simulink library "SERGIOarm"  (Simulink 7.9)
settings: Solver=ode45  StartTime=0.0  StopTime=10.0  RelTol=1e-3
undefined symbols (not defined in the file or in its folder): DiscIntNeverNeededParam
settings Model: Creator=root  LastModifiedBy=root

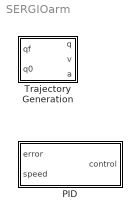
== system SERGIOarm ==
  PID : Subsystem  mask(PID Controller with anti wind-up){Kc=0, Ki=0, Kd=0, uplim=0, lowlim=0, Ts=0}
      mask prompts: Kc "P gain"; Ki "I gain"; Kd "D gain"; uplim "Integrator Upper Limit"; lowlim "Integrator Low Limit"; Ts "Sampling time (for integrator)"
      mask help: Outputs a control effort based on position error (error) and speed error (speed).
  Trajectory Generation : Subsystem  mask(Trajectory Generation){Vmax=0, Amax=0, dif_in=0}
      mask prompts: Vmax "Maximum Velocity"; Amax "Maximum Acceleration"; dif_in "Minimum Setpoint Change"
      mask help: Outputs setpoints (q) based on the starting point (q0) and end point (qf). The setpoints follow a fastest trajectory under the constraints of maximum velocity and maximum acceleration. Only outputs a trajectory if the setpoint change is more than the Minimum Setpoint Change variabele, in order to prevent trajectory generation for small deviations from the current setpoint.

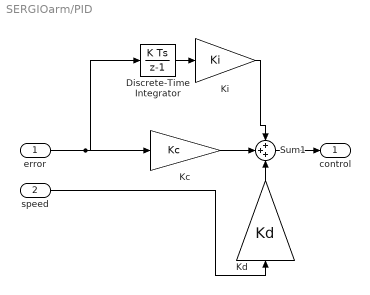
== system SERGIOarm/PID ==
  error : Inport
  speed : Inport  Port=2
  Discrete-Time Integrator : DiscreteIntegrator  SampleTime=Ts  LimitOutput=on  UpperSaturationLimit=uplim  LowerSaturationLimit=lowlim  ICPrevOutput=DiscIntNeverNeededParam  ICPrevScaledInput=DiscIntNeverNeededParam
  Kc : Gain  Gain=Kc
  Kd : Gain  Gain=Kd
  Ki : Gain  Gain=Ki
  Sum1 : Sum  Inputs=+++
  control : Outport
  wires:
  Kc/1 -> Sum1/2
  Kd/1 -> Sum1/3
  Ki/1 -> Sum1/1
  Discrete-Time Integrator/1 -> Ki/1
  error/1 -> Discrete-Time Integrator/1, Kc/1
  speed/1 -> Kd/1
  Sum1/1 -> control/1

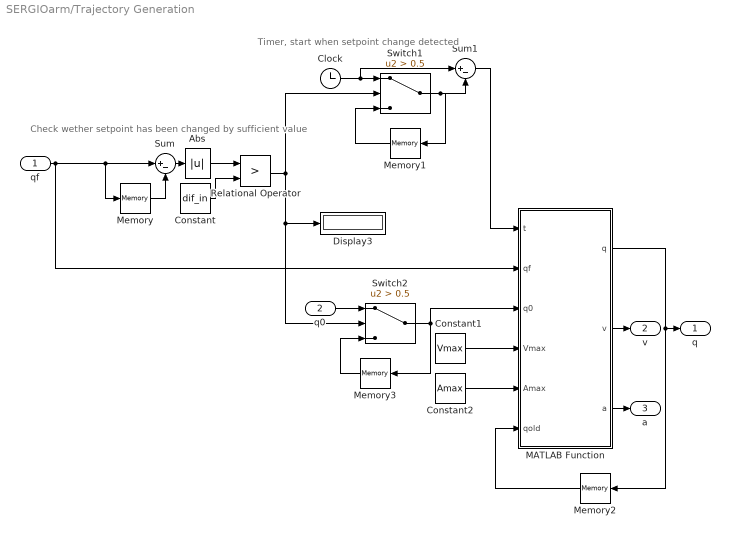
== system SERGIOarm/Trajectory Generation ==
  note: Timer, start when setpoint change detected
  note: Check wether setpoint has been changed
      | by sufficient value
  qf : Inport
  q0 : Inport  Port=2
  Abs : Abs
  Clock : Clock
  Constant : Constant  Value=dif_in
  Constant1 : Constant  Value=Vmax
  Constant2 : Constant  Value=Amax
  Display3 : Display
  MATLAB Function : MATLAB Function  TreatAsAtomicUnit=on
  Memory{,1..3} (4 alike) : Memory
  Relational Operator : RelationalOperator  Operator=>  OutDataTypeStr=boolean
  Sum : Sum  Inputs=|+-
  Sum1 : Sum  Inputs=|+-
  Switch1 : Switch  Criteria=u2 > Threshold  Threshold=0.5
  Switch2 : Switch  Criteria=u2 > Threshold  Threshold=0.5
  q : Outport
  v : Outport  Port=2
  a : Outport  Port=3
  wires:
  qf/1 -> MATLAB Function/2(qf), Sum/1, Memory/1
  Memory/1 -> Sum/2
  Sum/1 -> Abs/1
  Constant/1 -> Relational Operator/2
  Relational Operator/1 -> Switch1/2, Display3/1, Switch2/2
  Switch1/1 -> Memory1/1, Sum1/2
  Memory1/1 -> Switch1/3
  Clock/1 -> Switch1/1, Sum1/1
  Sum1/1 -> MATLAB Function/1(t)
  MATLAB Function/1(q) -> q/1, Memory2/1
  Constant1/1 -> MATLAB Function/4(Vmax)
  Constant2/1 -> MATLAB Function/5(Amax)
  Memory2/1 -> MATLAB Function/6(qold)
  Abs/1 -> Relational Operator/1
  q0/1 -> Switch2/1
  Switch2/1 -> Memory3/1, MATLAB Function/3(q0)
  Memory3/1 -> Switch2/3
  MATLAB Function/2(v) -> v/1
  MATLAB Function/3(a) -> a/1

== matlab function Trajectory Generation/MATLAB Function ==
  data: t input double; qf input double; q output double; q0 input double; Vmax input double; Amax input double; qold input double; v output double; a output double
function [q,v,a]  = LSPBfunc(t,qf,q0,Vmax,Amax,qold)

if(qf<0)
    qf = -qf;
    q0 = -q0;
    qneg = 1;
else
    qneg = 0;
end

tb = Vmax/Amax;

qtb = tb^2*Amax/2;
qleft = abs(qf-q0)-2*qtb;
tleft = qleft/Vmax;


if(tleft >= 0)
    tf = 2*tb+tleft;
    
    if(qf>q0)
        if(t<=tb)
            q = q0+t^2*Amax/2;
            v = Amax*t;
            a = Amax;
        elseif((t > tb) && (t <= tf-tb))
            q = (qf+q0-Vmax*tf)/2+Vmax*t;
            v = Vmax;
            a = 0;
        else
            q = qf-Amax*tf^2/2+Amax*tf*t-Amax/2*t^2;
            v = Amax*(tf-t);
            a = -Amax;
        end
    else
        if(t<=tb)
            q = q0-t^2*Amax/2;
            v = -Amax*t;
            a = -Amax;
        elseif((t > tb) && (t <= tf-tb))
            q = (qf+q0+Vmax*tf)/2-Vmax*t;
            v = -Vmax;
            a = 0;
        else
            q = qf+Amax*tf^2/2-Amax*tf*t+Amax/2*t^2;
            v = Amax*(t-tf);
            a = Amax;
        end
    end
else
    ts = sqrt(abs(qf-q0)/Amax);
    tf = 2*ts;
    if(qf>q0)
        if(t<=ts)
            q = q0+t^2*Amax/2;
            v = Amax*t;
            a = Amax;
        else
            q = qf-Amax*tf^2/2+Amax*tf*t-Amax/2*t^2;
            v = Amax*(tf-t);
            a = -Amax;
        end
    else
        if(t<=ts)
            q = q0-t^2*Amax/2;
            v = -Amax*t;
            a = -Amax;
        else
            q = qf+Amax*tf^2/2-Amax*tf*t+Amax/2*t^2;
            v = Amax*(t-tf);
            a = Amax;
        end
    end
end


if(qneg)
    q = -q;
    v = -v;
    a = -a;
end
if(t>tf)
    q = qold;
end


end
